simulink model "Auto_landing"  (R2019a)
settings: Solver=VariableStepAuto  StartTime=0.0  StopTime=500  RelTol=1e-3  EnableMultiTasking=on
values from neighbouring files (symbols this model uses):
  A1 = [X_u+X_T_u X_alpha 0 -g*cos(theta_1) ... (first row only)    [Cesna182_flight_dy.m]
  B1 = [X_de 0 ... (first row only)    [Cesna182_flight_dy.m]
  C1 = [1 0 0 0 ... (first row only)    [Cesna182_flight_dy.m]
  D1 = [0 0 ... (first row only)    [Cesna182_flight_dy.m]
  U_1 = 67.08648    [Cesna182_flight_dy.m]
libraries: simulink x1
settings Model: Creator=felip  LastModifiedBy=yuril
settings DataIOCC: ReturnWorkspaceOutputs=off
settings OptimizationCC: LifeSpan=inf
settings DebuggingCC: SFUnexpectedBacktrackingDiag=warning  SFNoUnconditionalDefaultTransitionDiag=warning  ArithmeticOperatorsInVariantConditions=warning
settings SFSimCC: SimUseLocalCustomCode=off
settings RTWCC: RTWUseLocalCustomCode=off
settings CodeAppCC: StateflowObjectComments=on
settings GRTTargetCC: TargetLangStandard=C89/C90 (ANSI)  GeneratePreprocessorConditionals=Disable all
settings ConfigComp: CovMetricSettings=dw  CovHtmlReporting=on  CovSaveCumulativeToWorkspaceVar=on  CovSaveSingleToWorkspaceVar=on  CovExternalEMLEnable=off

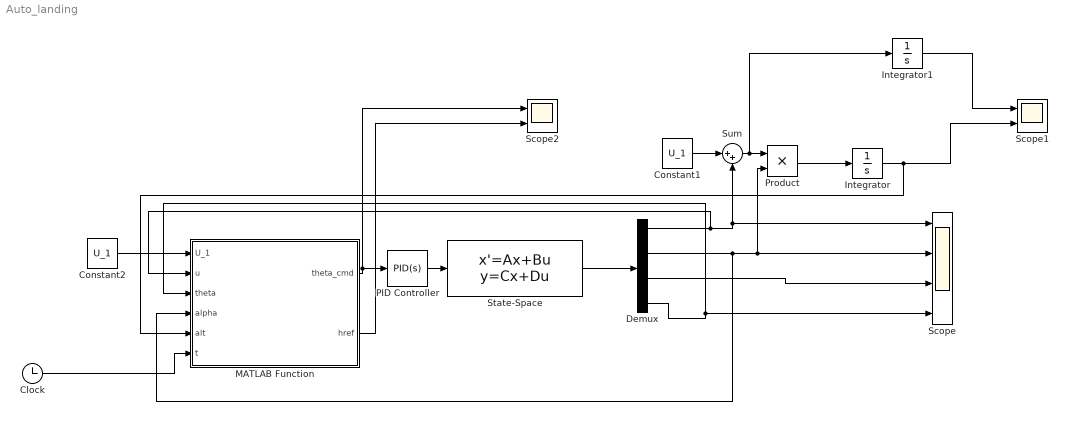
== system Auto_landing ==
  Clock : Clock
      settings: Decimation=100
  Constant1 : Constant  Value=U_1
  Constant2 : Constant  Value=U_1
  Demux : Demux
  Integrator : Integrator  InitialCondition=100
  Integrator1 : Integrator
  MATLAB Function : MATLAB Function  TreatAsAtomicUnit=on
  PID Controller : simulink/Continuous/PID Controller  Controller=PID  Form=Parallel  TimeDomain=Continuous-time  SampleTime=-1  IntegratorMethod=Forward Euler  FilterMethod=Forward Euler  ControllerParametersSource=internal  P=-0.00208689038935795  I=-9.47854235710142e-05  D=0.000110510959538448  UseFilter=on  N=18.8840129347705  TunerSelectOption=Transfer Function Based (PID Tuner App)  InitialConditionSource=internal  InitialConditionForIntegrator=0  InitialConditionForFilter=0  DifferentiatorICPrevScaledInput=0  ExternalReset=none  TrackingMode=off  Kt=1  LimitOutput=off  UpperSaturationLimit=inf  LowerSaturationLimit=-inf  LinearizeAsGain=on  AntiWindupMode=none  Kb=1  POutMin=[]  POutMax=[]  IOutMin=[]  IOutMax=[]  DOutMin=[]  DOutMax=[]  NOutMin=[]  NOutMax=[]  SumOutMin=[]  SumOutMax=[]  SaturationOutMin=[]  SaturationOutMax=[]  PParamMin=[]  PParamMax=[]  IParamMin=[]  IParamMax=[]  DParamMin=[]  DParamMax=[]  NParamMin=[]  NParamMax=[]  KbParamMin=[]  KbParamMax=[]  KtParamMin=[]  KtParamMax=[]  KbOutMin=[]  KbOutMax=[]  KtOutMin=[]  KtOutMax=[]  IntegratorOutMin=[]  IntegratorOutMax=[]  FilterOutMin=[]  FilterOutMax=[]  SumI1OutMin=[]  SumI1OutMax=[]  SumI2OutMin=[]  SumI2OutMax=[]  SumI3OutMin=[]  SumI3OutMax=[]  SumI4OutMin=[]  SumI4OutMax=[]  SumDOutMin=[]  SumDOutMax=[]  DifferentiatorOutMin=[]  DifferentiatorOutMax=[]  FilterDiffOutCoefMin=[]  FilterDiffOutCoefMax=[]  ReciprocalOutMin=[]  ReciprocalOutMax=[]  SumDenOutMin=[]  SumDenOutMax=[]  SumNumOutMin=[]  SumNumOutMax=[]  DivideOutMin=[]  DivideOutMax=[]  IntegratorContinuousStateAttributes=''  IntegratorStateMustResolveToSignalObject=off  IntegratorRTWStateStorageClass=Auto  FilterContinuousStateAttributes=''  FilterStateMustResolveToSignalObject=off  FilterRTWStateStorageClass=Auto  ParallelPVariant=InternalParameters  IdealPVariant=Disabled  IVariant=InternalParameters  DVariant=InternalParameters  IntegratorVariant=Continuous  SatVariant=Disabled  AWVariant=Passthrough  PCopyVariant=Disabled  TRVariant=Disabled  FdbkBlocksVariant=Forward  IdealPFdbkVariant=Disabled  SatFdbkVariant=Disabled  DerivativeFilterVariant=ContFilter  NVariant=InternalParameters  NCopyVariant=Disabled  FilterICVariant=InternalICsFilter  IntegratorICVariant=InternalICs  ExternalResetVariant=Disabled  TRSumVariant=Passthrough  SumFdbkVariant=Disabled  SumVariant=Sum_PID
  Product : Product
  Scope : Scope  NumInputPorts=4
  Scope1 : Scope  NumInputPorts=2
  Scope2 : Scope  NumInputPorts=2
  State-Space : StateSpace  A=A1  B=B1(:,1)  C=C1  D=D1(:,1)  InitialCondition=0
  Sum : Sum  Inputs=|++
  wires:
  State-Space/1 -> Demux/1
  Demux/4 -> MATLAB Function/3(theta), Scope/4
  Demux/3 -> Scope/3
  PID Controller/1 -> State-Space/1
  Demux/1 -> MATLAB Function/2(u), Sum/2, Scope/1
  Demux/2 -> MATLAB Function/4(alpha), Product/2, Scope/2
  Product/1 -> Integrator/1
  MATLAB Function/1(theta_cmd) -> PID Controller/1, Scope2/1
  Constant1/1 -> Sum/1
  Sum/1 -> Integrator1/1, Product/1
  Constant2/1 -> MATLAB Function/1(U_1)
  Clock/1 -> MATLAB Function/6(t)
  MATLAB Function/2(href) -> Scope2/2
  Integrator1/1 -> Scope1/1
  Integrator/1 -> MATLAB Function/5(alt), Scope1/2

== matlab function Auto_landing/MATLAB Function ==
  data: U_1 input; u input; theta input; alpha input; alt input; theta_cmd output; t input; href output
function [theta_cmd,href] = fcn(U_1,u,theta,alpha,alt,t)
h0 = 100;
Dhor = 1000;
tau = Dhor/U_1;
href = h0*exp(-t/tau);
gamma_ref = (href-alt)/((U_1+u)*0.01);

%h_dot = -h/tau;

theta_d = gamma_ref+alpha;

theta_cmd = theta_d - theta;

end
